simulink model "sandbox"  (R2019a)
settings: Solver=VariableStepAuto  StartTime=0.0  StopTime=10  RelTol=1e-3
undefined symbols (not defined in the file): GHC_B, IHC_B, ILC_B, IPT_B
settings Model: Creator=rache  LastModifiedBy=rache

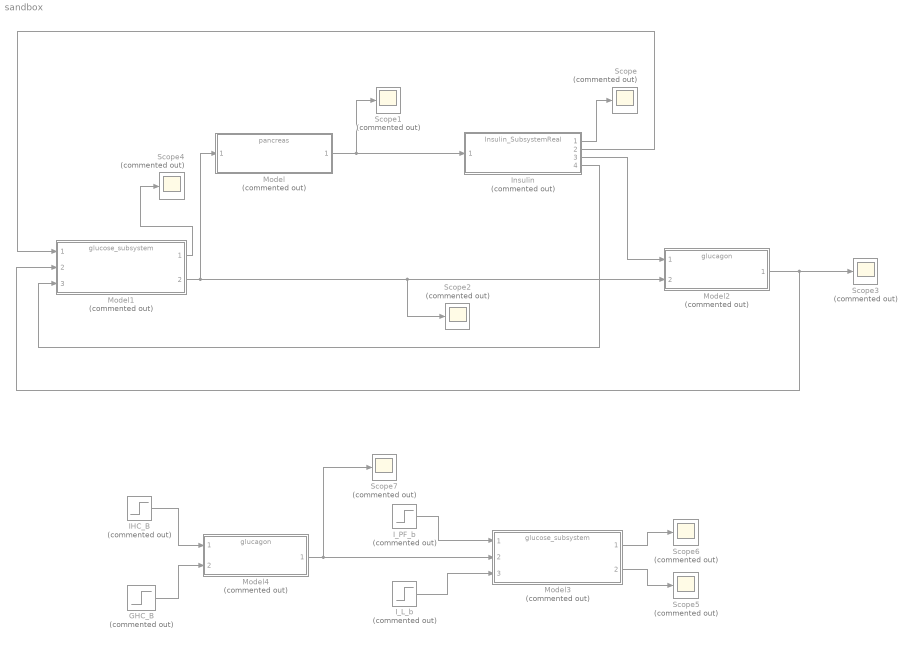
== system sandbox ==
  GHC_B : Step  Commented=on  After=GHC_B  SampleTime=0.1
  IHC_B : Step  Commented=on  After=IHC_B  SampleTime=0.1
  I_L_b : Step  Commented=on  After=ILC_B  SampleTime=0.1
  I_PF_b : Step  Commented=on  After=IPT_B  SampleTime=0.1
  Insulin : ModelReference  Commented=on  ModelNameDialog=Insulin_SubsystemReal  SimulationMode=Normal  ModelReferenceVersion=1.40
  Model : ModelReference  Commented=on  ModelNameDialog=pancreas  SimulationMode=Normal  ModelReferenceVersion=1.16
  Model1 : ModelReference  Commented=on  ModelNameDialog=glucose_subsystem  SimulationMode=Normal  ModelReferenceVersion=1.50
  Model2 : ModelReference  Commented=on  ModelNameDialog=glucagon  SimulationMode=Normal  ModelReferenceVersion=1.11
  Model3 : ModelReference  Commented=on  ModelNameDialog=glucose_subsystem  SimulationMode=Normal  ModelReferenceVersion=1.63
  Model4 : ModelReference  Commented=on  ModelNameDialog=glucagon  SimulationMode=Normal  ModelReferenceVersion=1.11
  Scope{,1..7} (8 alike) : Scope  Commented=on
  wires:
  Model/1 -> Scope1/1, Insulin/1
  Insulin/1 -> Scope/1
  Model1/2 -> Model2/2, Scope2/1, Model/1
  Insulin/3 -> Model2/1
  Model2/1 -> Scope3/1, Model1/2
  Insulin/2 -> Model1/1
  Insulin/4 -> Model1/3
  Model1/1 -> Scope4/1
  Model3/2 -> Scope5/1
  I_L_b/1 -> Model3/3
  I_PF_b/1 -> Model3/1
  Model4/1 -> Model3/2, Scope7/1
  Model3/1 -> Scope6/1
  IHC_B/1 -> Model4/1
  GHC_B/1 -> Model4/2
